simulink model "oscillator_converge"  (R2023b)
settings: Solver=VariableStepAuto  StartTime=0.0  StopTime=100  RelTol=1e-3
settings Model: Creator=awcm9  LastModifiedBy=awcm9

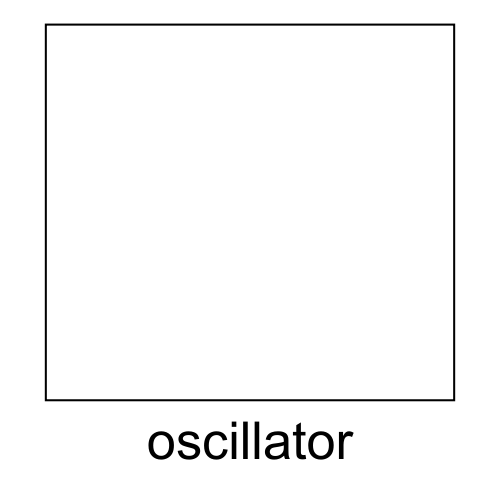
[thumbnail: Simulink's stored preview of the top-level diagram]
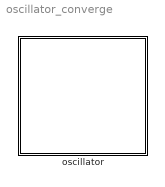
== system oscillator_converge ==
  oscillator : Subsystem

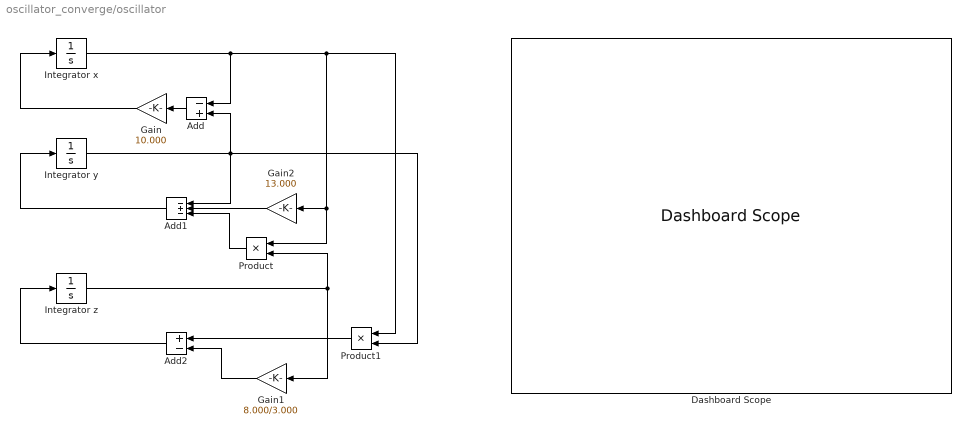
== system oscillator_converge/oscillator ==
  Add : Sum  Inputs=-+
  Add1 : Sum  Inputs=-+-
  Add2 : Sum  Inputs=+-
  Dashboard Scope : DashboardScope  ShowInitialText=off  TimeSpan=5  Ymin=-50  Ymax=50  ScaleAtStop=off
  Gain : Gain  Gain=10.000
  Gain1 : Gain  Gain=8.000/3.000
  Gain2 : Gain  Gain=13.000
  Integrator x : Integrator  InitialCondition=1
  Integrator y : Integrator
  Integrator z : Integrator
  Product : Product
  Product1 : Product
  wires:
  Add2/1 -> Integrator z/1
  Gain1/1 -> Add2/2
  Product1/1 -> Add2/1
  Add1/1 -> Integrator y/1
  Product/1 -> Add1/3
  Gain2/1 -> Add1/2
  Gain/1 -> Integrator x/1
  Integrator z/1 -> Product/2, Gain1/1
  Add/1 -> Gain/1
  Integrator y/1 -> Add/2, Add1/1, Product1/2
  Integrator x/1 -> Gain2/1, Product/1, Product1/1, Add/1
